simulink model "TcpIP_model"  (Simulink 9.1)
settings: Solver=ode45  StartTime=0  StopTime=5  FixedStep=TSTEP  RelTol=1e-3  EnableMultiTasking=on
PreLoadFcn:
  | cd extensions\simulink\pt_center_diff
  | Run_ft4wd_eclass
  | lsd_parameta_eclass
  | cd ..\..\..
libraries: Solver_SF x1
settings Model: Creator=ywata  LastModifiedBy=xiaoyu  ExtModeTrigMode=oneshot  ExtModeArmWhenConnect=off
settings SolverCC: AlgebraicLoopSolver=LineSearch
settings DataIOCC: SignalLoggingSaveFormat=ModelDataLogs  SaveOutput=off  SaveTime=off  SignalLoggingName=sigsOut
settings OptimizationCC: BooleanDataType=off
settings DebuggingCC: SaveWithParameterizedLinksMsg=none  SignalResolutionControl=TryResolveAllWithWarning  MultiTaskDSMMsg=warning  MultiTaskCondExecSysMsg=none  FcnCallInpInsideContextMsg=warning  StateNameClashWarn=warning
settings HardwareCC: TargetBitPerPointer=64  TargetBitPerSizeT=64  TargetBitPerPtrDiffT=64  TargetLongLongMode=on  TargetIntDivRoundTo=Zero  TargetEndianess=LittleEndian  TargetWordSize=64  TargetHWDeviceType=MATLAB Host  ProdEqTarget=off
settings GRTTargetCC: TargetFcnLib=ansi_tfl_tmw.mat  ModelReferenceCompliant=off  MatFileLogging=off

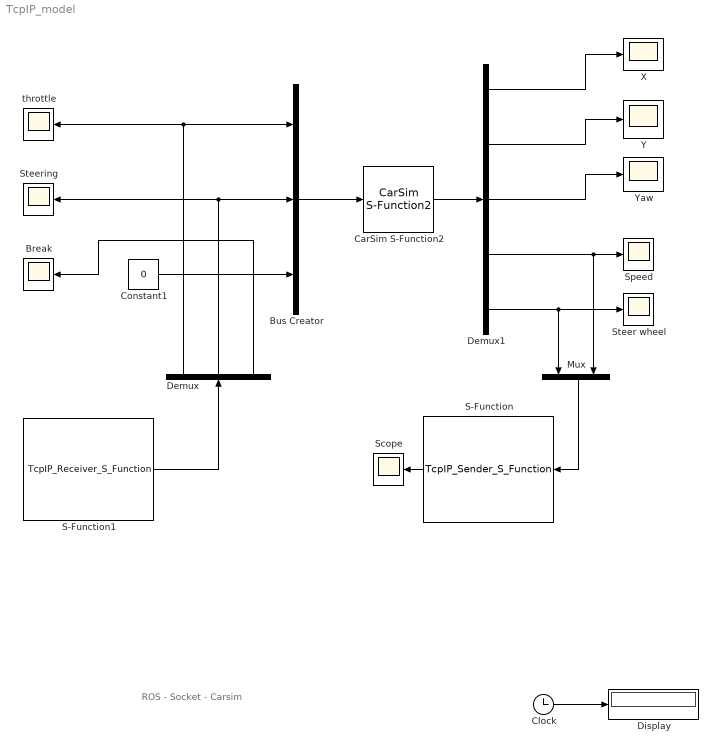
== system TcpIP_model ==
  note: ROS - Socket - Carsim
  Break : Scope
  Bus Creator : BusCreator  Inputs=3
  CarSim S-Function2 : Solver_SF/CarSim S-Function2  Priority=1  VehicleCode=i_s  SIMFILE=simfile.sim
      settings: AttributesFormatString=Vehicle Code: %<VehicleCode>
  Clock : Clock
  Constant1 : Constant  Value=0
  Demux : Demux  Outputs=3
  Demux1 : Demux  Outputs=5
  Display : Display
  Mux : Mux  Inputs=2
  S-Function : S-Function  FunctionName=TcpIP_Sender_S_Function  SFunctionDeploymentMode=off  EnableBusSupport=off
  S-Function1 : S-Function  FunctionName=TcpIP_Receiver_S_Function  SFunctionDeploymentMode=off  EnableBusSupport=off
  Scope : Scope
  Speed : Scope
  Steer wheel : Scope
  Steering : Scope
  X : Scope
  Y : Scope
  Yaw : Scope
  throttle : Scope
  wires:
  Clock/1 -> Display/1
  Demux1/4 -> Mux/2, Speed/1
  Demux1/3 -> Yaw/1
  Demux1/2 -> Y/1
  Demux1/1 -> X/1
  Demux1/5 -> Mux/1, Steer wheel/1
  CarSim S-Function2/1 -> Demux1/1
  Bus Creator/1 -> CarSim S-Function2/1
  Constant1/1 -> Bus Creator/3
  S-Function/1 -> Scope/1
  Mux/1 -> S-Function/1
  S-Function1/1 -> Demux/1
  Demux/1 -> throttle/1, Bus Creator/1
  Demux/2 -> Bus Creator/2, Steering/1
  Demux/3 -> Break/1
